simulink model "LFC"  (R2014a)
settings: Solver=ode45  StartTime=0.0  StopTime=60  RelTol=1e-3
libraries: cstblocks x10
settings Model: Creator=Divya M  LastModifiedBy=Divya M

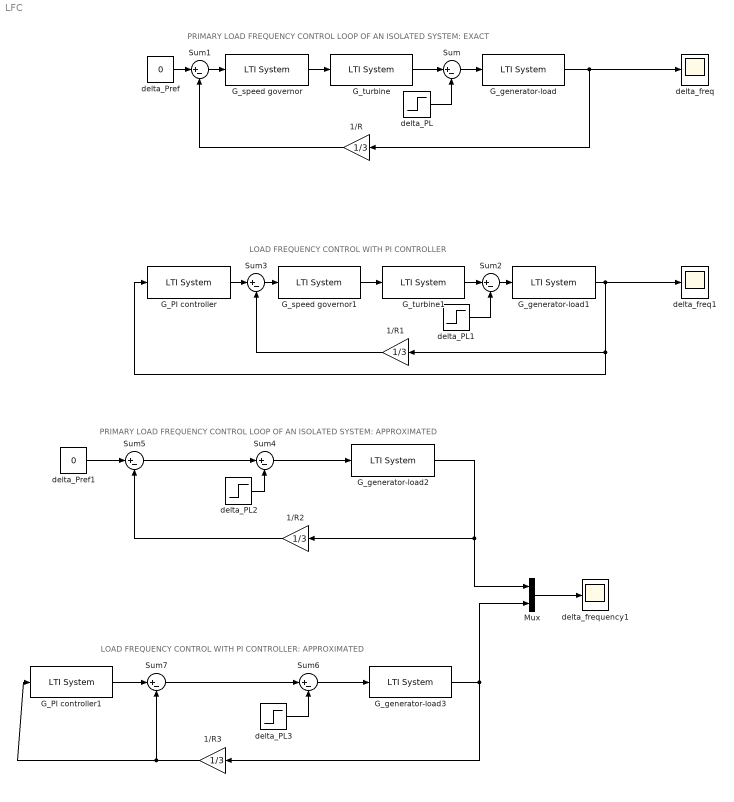
== system LFC ==
  note: PRIMARY LOAD FREQUENCY CONTROL LOOP OF AN ISOLATED SYSTEM: EXACT
  note: LOAD FREQUENCY CONTROL WITH PI CONTROLLER
  note: PRIMARY LOAD FREQUENCY CONTROL LOOP OF AN ISOLATED SYSTEM: APPROXIMATED
  note: LOAD FREQUENCY CONTROL WITH PI CONTROLLER: APPROXIMATED
  1/R{,1..3} (4 alike) : Gain  Gain=1/3
  G_PI controller : cstblocks/LTI System  sys=tf(-.03,[1 0])  IC=[]
  G_PI controller1 : cstblocks/LTI System  sys=tf(-0.09,[1 0])  IC=[]
  G_generator-load{,1..3} (4 alike) : cstblocks/LTI System  sys=tf(100,[20 1])  IC=[]
  G_speed governor : cstblocks/LTI System  sys=tf(10,[0.4 1])  IC=[]
  G_speed governor1 : cstblocks/LTI System  sys=tf(10,[0.4 1])  IC=[]
  G_turbine : cstblocks/LTI System  sys=tf(0.1,[0.5 1])  IC=[]
  G_turbine1 : cstblocks/LTI System  sys=tf(0.1,[0.5 1])  IC=[]
  Mux : Mux  Inputs=2
  Sum{,1..7} (8 alike) : Sum  Inputs=|+-
  delta_PL{,1..3} (4 alike) : Step  After=0.01  SampleTime=0
  delta_Pref : Constant  Value=0
  delta_Pref1 : Constant  Value=0
  delta_freq : Scope
      settings: YMin=-0.05  YMax=0.005  SaveName=ScopeData2
  delta_freq1 : Scope
      settings: YMin=-0.05  YMax=0.005
  delta_frequency1 : Scope
      settings: YMin=-0.05  YMax=0.01
  wires:
  delta_Pref/1 -> Sum1/1
  Sum1/1 -> G_speed governor/1
  G_speed governor/1 -> G_turbine/1
  G_turbine/1 -> Sum/1
  Sum/1 -> G_generator-load/1
  G_generator-load/1 -> delta_freq/1, 1/R/1
  delta_PL/1 -> Sum/2
  1/R/1 -> Sum1/2
  Sum3/1 -> G_speed governor1/1
  G_speed governor1/1 -> G_turbine1/1
  G_turbine1/1 -> Sum2/1
  Sum2/1 -> G_generator-load1/1
  G_generator-load1/1 -> delta_freq1/1, G_PI controller/1, 1/R1/1
  delta_PL1/1 -> Sum2/2
  1/R1/1 -> Sum3/2
  G_PI controller/1 -> Sum3/1
  delta_Pref1/1 -> Sum5/1
  Sum4/1 -> G_generator-load2/1
  G_generator-load2/1 -> Mux/1, 1/R2/1
  delta_PL2/1 -> Sum4/2
  1/R2/1 -> Sum5/2
  Sum7/1 -> Sum6/1
  Sum6/1 -> G_generator-load3/1
  delta_PL3/1 -> Sum6/2
  1/R3/1 -> G_PI controller1/1, Sum7/2
  G_PI controller1/1 -> Sum7/1
  Sum5/1 -> Sum4/1
  Mux/1 -> delta_frequency1/1
  G_generator-load3/1 -> 1/R3/1, Mux/2
